simulink model "MPG_MG_PLL_orig"  (R2021b)
settings: Solver=VariableStepAuto  StartTime=0.0  StopTime=1  RelTol=1e-3
model workspace (MAT data in the model file):
  Ts : Simulink.Parameter (value not decoded)
  secondary_on : Simulink.Parameter (value not decoded)
values from neighbouring files (symbols this model uses):
  A = zeros(4,4)    [MPC_MG_script_raw_dmpc.m]    (also in MPG_MG_July.m = [0 1 1 1; 1 0 0 0; 1 0 0 0; 1 0 0 0]; MPG_MG_freq_script.m = ones(4) - eye(4); Script.m = [0 1 1 1 ; 1 0 1 1 ; 1 1 0 1 ; 1 1 1 0])
  C_f = 50e-6    (= 5e-05)    [Four_DG_MG_PrimaryOnlyScript.m]    (also in MPC_MG_script.m; MPC_MG_script_raw_dmpc.m; MPC_MG_secondary_script.m; MPG_MG_July.m)
  f_c = 5000    [Four_DG_MG_PrimaryOnlyScript.m]    (also in MPC_MG_script.m = 40000; MPC_MG_script_raw_dmpc.m = 40000; MPC_MG_secondary_script.m = 40000; MPG_MG_July.m = 50000)
  kL = 1e-5    (= 1e-05)    [Four_DG_MG_PrimaryOnlyScript.m]    (also in MPC_MG_script.m = 1e-08; MPC_MG_script_raw_dmpc.m = 1e-08; MPC_MG_secondary_script.m = 1e-07; MPG_MG_July.m = 1e-07)
  L_f = 1.35e-3    (= 0.00135)    [Four_DG_MG_PrimaryOnlyScript.m]    (also in MPC_MG_script.m; MPC_MG_script_raw_dmpc.m; MPC_MG_secondary_script.m; MPG_MG_July.m)
  L_in1 = 0.35e-3    (= 0.00035)    [Four_DG_MG_PrimaryOnlyScript.m]    (also in MPC_MG_script.m; MPC_MG_script_raw_dmpc.m; MPC_MG_secondary_script.m; MPG_MG_July.m)
  L_in2 = 0.35e-3    (= 0.00035)    [Four_DG_MG_PrimaryOnlyScript.m]    (also in MPC_MG_script.m; MPC_MG_script_raw_dmpc.m; MPC_MG_secondary_script.m; MPG_MG_July.m)
  L_in4 = 0.35e-3    (= 0.00035)    [Four_DG_MG_PrimaryOnlyScript.m]    (also in MPC_MG_script.m; MPC_MG_script_raw_dmpc.m; MPC_MG_secondary_script.m; MPG_MG_July.m)
  lambda1 = [30000 50000 90000 50000]'    [MPC_MG_script_raw_dmpc.m]    (also in MPG_MG_July.m = [4 4 4 4]'; MPG_MG_freq_script.m = [3 3 3 3]'; Script.m = [1 1 1 1]')
  lambda2 = [5 6 7 6]'    [MPC_MG_script_raw_dmpc.m]    (also in MPG_MG_July.m = [0.5e-2 0.5e-2 0.5e-2 0.5e-2]'; MPG_MG_freq_script.m = [1.1 1.9 1.5 1.2]'; Script.m = [0.8e-2 0.8e-2 0.8e-2 0.8e-2]')
  lambda3 = [80000 80000 900000 80000]'    [MPC_MG_script_raw_dmpc.m]    (also in MPG_MG_July.m = [1e-3 1e-3 1e-3 1e-3]'; MPG_MG_freq_script.m = [9e-4 1.2e-2 3e-3 3e-3]'; Script.m = [1.5e-3 1.5e-3 1.5e-3 1.5e-3]')
  LD_ref1 = 800e-6    (= 0.0008)    [Four_DG_MG_PrimaryOnlyScript.m]    (also in MPC_MG_script.m = 0.0003; MPC_MG_script_raw_dmpc.m = 0.0003; MPC_MG_secondary_script.m = 0.0001; MPG_MG_July.m = 0.0004)
  lo_co = 0.2    [Four_DG_MG_PrimaryOnlyScript.m]    (also in MPC_MG_script.m = 0.05; MPC_MG_script_raw_dmpc.m; MPC_MG_secondary_script.m = 0.08; MPG_MG_July.m = 0.15)
  m_p1 = 9.4e-5/droopDivide    (= 9.4e-05)    [Four_DG_MG_PrimaryOnlyScript.m]    (also in MPC_MG_script.m; MPC_MG_script_raw_dmpc.m; MPC_MG_secondary_script.m; MPG_MG_July.m)
  m_p2 = 9.4e-5/droopDivide    (= 9.4e-05)    [Four_DG_MG_PrimaryOnlyScript.m]    (also in MPC_MG_script.m; MPC_MG_script_raw_dmpc.m; MPC_MG_secondary_script.m; MPG_MG_July.m)
  m_p3 = 12.5e-5/droopDivide    (= 0.000125)    [Four_DG_MG_PrimaryOnlyScript.m]    (also in MPC_MG_script.m; MPC_MG_script_raw_dmpc.m; MPC_MG_secondary_script.m; MPG_MG_July.m)
  m_p4 = 12.5e-5/droopDivide    (= 0.000125)    [Four_DG_MG_PrimaryOnlyScript.m]    (also in MPC_MG_script.m; MPC_MG_script_raw_dmpc.m; MPC_MG_secondary_script.m; MPG_MG_July.m)
  N = 3    [MPG_MG_July.m]    (also in MPG_MG_freq_script.m = 2; Script.m = 5)
  n_q1 = 1.3e-3/droopDivide2    (= 0.00013)    [Four_DG_MG_PrimaryOnlyScript.m]    (also in MPC_MG_script.m; MPC_MG_script_raw_dmpc.m; MPC_MG_secondary_script.m; MPG_MG_July.m)
  n_q2 = 1.3e-3/droopDivide2    (= 0.00013)    [Four_DG_MG_PrimaryOnlyScript.m]    (also in MPC_MG_script.m; MPC_MG_script_raw_dmpc.m; MPC_MG_secondary_script.m; MPG_MG_July.m)
  n_q4 = 1.5e-3/droopDivide2    (= 0.00015)    [Four_DG_MG_PrimaryOnlyScript.m]    (also in MPC_MG_script.m; MPC_MG_script_raw_dmpc.m; MPC_MG_secondary_script.m; MPG_MG_July.m)
  Pmax = [45e3 45e3 37e3 37e3]'    [MPG_MG_July.m]    (also in MPG_MG_freq_script.m; Script.m)
  R_f = 0.1    [Four_DG_MG_PrimaryOnlyScript.m]    (also in MPC_MG_script.m; MPC_MG_script_raw_dmpc.m; MPC_MG_secondary_script.m; MPG_MG_July.m)
  R_in1 = 0.03    [Four_DG_MG_PrimaryOnlyScript.m]    (also in MPC_MG_script.m; MPC_MG_script_raw_dmpc.m; MPC_MG_secondary_script.m; MPG_MG_July.m)
  R_in2 = 0.03    [Four_DG_MG_PrimaryOnlyScript.m]    (also in MPC_MG_script.m; MPC_MG_script_raw_dmpc.m; MPC_MG_secondary_script.m; MPG_MG_July.m)
  R_in4 = 0.03    [Four_DG_MG_PrimaryOnlyScript.m]    (also in MPC_MG_script.m; MPC_MG_script_raw_dmpc.m; MPC_MG_secondary_script.m; MPG_MG_July.m)
  time_thresh = 0.6    [Four_DG_MG_PrimaryOnlyScript.m]    (also in MPC_MG_script_raw_dmpc.m = 1.5; MPC_MG_secondary_script.m = 2; MPG_MG_July.m = 0.5; MPG_MG_freq_script.m = 0.5)
  Ts = 10e-6    (= 1e-05)    [Four_DG_MG_PrimaryOnlyScript.m]    (also in MPC_MG_script.m; MPC_MG_script_raw_dmpc.m; MPC_MG_secondary_script.m; MPG_MG_July.m)
  Tsamp = 0.1    [MPG_MG_July.m]    (also in MPG_MG_freq_script.m; Script.m)
  V_nom = 220*sqrt(2)    [Four_DG_MG_PrimaryOnlyScript.m]    (also in MPC_MG_script.m; MPC_MG_script_raw_dmpc.m; MPC_MG_secondary_script.m; MPG_MG_July.m)
  Vdc = 600    [Four_DG_MG_PrimaryOnlyScript.m]    (also in MPC_MG_script.m; MPC_MG_script_raw_dmpc.m; MPC_MG_secondary_script.m; MPG_MG_July.m)
  w_c_high = 2*pi*50    (= 314.159265359)    [Four_DG_MG_PrimaryOnlyScript.m]    (also in MPC_MG_script.m; MPC_MG_script_raw_dmpc.m; MPC_MG_secondary_script.m; MPG_MG_July.m)
  w_nom = 2*pi*50    (= 314.159265359)    [Four_DG_MG_PrimaryOnlyScript.m]    (also in MPC_MG_script.m; MPC_MG_script_raw_dmpc.m; MPC_MG_secondary_script.m; MPG_MG_July.m)
undefined symbols (not defined in the file or in its folder): i
libraries: spsThreePhaseSeriesRLCBranchLib x18, spsabctodq0Lib x16, spsThreePhaseVIMeasurementLib x15, eeGeneralControl x15, dspswit3 x5, spsDCVoltageSourceLib x5, spsSeriesRLCBranchLib x5, spsTwoLevelConverterLib x5, slpidlib x5, spsAlphaBetaZerotodq0Lib x4, spsSecondOrderFilterLib x4, spsThreePhaseSeriesRLCLoadLib x2
(part 5 of 6)

== system MPG_MG_PLL_orig/Voltage Source Inverter 4/CDSC-PLL/DSC4/DSC_Beta ==
  Alpha : Inport
  Beta : Inport  Port=2
  Cos 2*pi/n : Subsystem
  Divide : Product  Inputs=*/
  Divide1 : Product  Inputs=*/
  Gain : Gain  Gain=1/2
  Product : Product
  Product1 : Product
  Sin 2*pi/n : Subsystem
  Sum1 : Sum  Inputs=+++
  T/n : Constant  Value=1/n
  T/n1 : Constant  Value=1/n
  Variable Transport Delay : VariableTransportDelay  VariableDelayType=Variable transport delay  MaximumDelay=10
  Variable Transport Delay1 : VariableTransportDelay  VariableDelayType=Variable transport delay  MaximumDelay=10
  Out : Outport  VectorParamsAs1DForOutWhenUnconnected=off
  wires:
  Gain/1 -> Out/1
  Sum1/1 -> Gain/1
  Beta/1 -> Variable Transport Delay/1, Sum1/1
  Alpha/1 -> Variable Transport Delay1/1
  Cos 2*pi/n/1(cos) -> Product/2
  Product/1 -> Sum1/2
  Variable Transport Delay/1 -> Product/1
  Variable Transport Delay1/1 -> Product1/1
  Product1/1 -> Sum1/3
  Sin 2*pi/n/1(sin) -> Product1/2
  T/n/1 -> Divide/1
  Divide/1 -> Variable Transport Delay/2
  [f_pll_c3] -> Divide/2
  T/n1/1 -> Divide1/1
  Divide1/1 -> Variable Transport Delay1/2
  [f_pll_c3] -> Divide1/2

== system MPG_MG_PLL_orig/Voltage Source Inverter 4/CDSC-PLL/DSC4/DSC_alpha ==
  Alpha : Inport
  Beta : Inport  Port=2
  Cos 2*pi/n : Subsystem
  Divide : Product  Inputs=*/
  Divide1 : Product  Inputs=*/
  Gain : Gain  Gain=1/2
  Product : Product
  Product1 : Product
  Sin 2*pi/n : Subsystem
  Sum1 : Sum  Inputs=++-
  T/n : Constant  Value=1/n
  T/n1 : Constant  Value=1/n
  Variable Transport Delay : VariableTransportDelay  VariableDelayType=Variable transport delay  MaximumDelay=10
  Variable Transport Delay1 : VariableTransportDelay  VariableDelayType=Variable transport delay  MaximumDelay=10
  Out : Outport  VectorParamsAs1DForOutWhenUnconnected=off
  wires:
  Sum1/1 -> Gain/1
  Gain/1 -> Out/1
  Sin 2*pi/n/1(sin) -> Product1/2
  Beta/1 -> Variable Transport Delay1/1
  Product1/1 -> Sum1/3
  Variable Transport Delay1/1 -> Product1/1
  Alpha/1 -> Variable Transport Delay/1, Sum1/1
  Variable Transport Delay/1 -> Product/1
  Product/1 -> Sum1/2
  Cos 2*pi/n/1(cos) -> Product/2
  T/n1/1 -> Divide/1
  Divide/1 -> Variable Transport Delay1/2
  [f_pll_c3] -> Divide/2
  T/n/1 -> Divide1/1
  Divide1/1 -> Variable Transport Delay/2
  [f_pll_c3] -> Divide1/2

== system MPG_MG_PLL_orig/Voltage Source Inverter 4/CDSC-PLL/DSC8/DSC_Beta ==
  Alpha : Inport
  Beta : Inport  Port=2
  Cos 2*pi/n : Subsystem
  Divide : Product  Inputs=*/
  Divide1 : Product  Inputs=*/
  Gain : Gain  Gain=1/2
  Product : Product
  Product1 : Product
  Sin 2*pi/n : Subsystem
  Sum1 : Sum  Inputs=+++
  T/n : Constant  Value=1/n
  T/n1 : Constant  Value=1/n
  Variable Transport Delay : VariableTransportDelay  VariableDelayType=Variable transport delay  MaximumDelay=10
  Variable Transport Delay1 : VariableTransportDelay  VariableDelayType=Variable transport delay  MaximumDelay=10
  Out : Outport  VectorParamsAs1DForOutWhenUnconnected=off
  wires:
  Sin 2*pi/n/1(sin) -> Product1/2
  Product1/1 -> Sum1/3
  Variable Transport Delay1/1 -> Product1/1
  Variable Transport Delay/1 -> Product/1
  Product/1 -> Sum1/2
  Cos 2*pi/n/1(cos) -> Product/2
  Alpha/1 -> Variable Transport Delay1/1
  Beta/1 -> Sum1/1, Variable Transport Delay/1
  Sum1/1 -> Gain/1
  Gain/1 -> Out/1
  T/n/1 -> Divide/1
  Divide/1 -> Variable Transport Delay/2
  [f_pll_c3] -> Divide/2
  T/n1/1 -> Divide1/1
  Divide1/1 -> Variable Transport Delay1/2
  [f_pll_c3] -> Divide1/2

== system MPG_MG_PLL_orig/Voltage Source Inverter 4/CDSC-PLL/DSC8/DSC_alpha ==
  Alpha : Inport
  Beta : Inport  Port=2
  Cos 2*pi/n : Subsystem
  Divide : Product  Inputs=*/
  Divide1 : Product  Inputs=*/
  Gain : Gain  Gain=1/2
  Product : Product
  Product1 : Product
  Sin 2*pi/n : Subsystem
  Sum1 : Sum  Inputs=++-
  T/n : Constant  Value=1/n
  T/n1 : Constant  Value=1/n
  Variable Transport Delay : VariableTransportDelay  VariableDelayType=Variable transport delay  MaximumDelay=10
  Variable Transport Delay1 : VariableTransportDelay  VariableDelayType=Variable transport delay  MaximumDelay=10
  Out : Outport  VectorParamsAs1DForOutWhenUnconnected=off
  wires:
  Cos 2*pi/n/1(cos) -> Product/2
  Product/1 -> Sum1/2
  Variable Transport Delay/1 -> Product/1
  Alpha/1 -> Variable Transport Delay/1, Sum1/1
  Variable Transport Delay1/1 -> Product1/1
  Product1/1 -> Sum1/3
  Beta/1 -> Variable Transport Delay1/1
  Sin 2*pi/n/1(sin) -> Product1/2
  Gain/1 -> Out/1
  Sum1/1 -> Gain/1
  T/n/1 -> Divide/1
  Divide/1 -> Variable Transport Delay/2
  [f_pll_c3] -> Divide/2
  T/n1/1 -> Divide1/1
  Divide1/1 -> Variable Transport Delay1/2
  [f_pll_c3] -> Divide1/2

== system MPG_MG_PLL_orig/Voltage Source Inverter 4/CDSC-PLL/SRF-PLL1/Al_Be_0 to dq0 ==
  Al_Be_0 : Inport
  wt : Inport  Port=2
  Fcn : Fcn  Expr=u[1]*cos(u[4]) + u[2]*sin(u[4])
  Fcn1 : Fcn  Expr=-u[1]*sin(u[4]) + u[2]*cos(u[4])
  Fcn2 : Fcn  Expr=u[3]
  Mux1 : Mux  Inputs=[3 1]
  Mux2 : Mux  Inputs=3
  dq0 : Outport  VectorParamsAs1DForOutWhenUnconnected=off
  wires:
  Mux1/1 -> Fcn/1, Fcn2/1, Fcn1/1
  Fcn1/1 -> Mux2/2
  wt/1 -> Mux1/2
  Mux2/1 -> dq0/1
  Al_Be_0/1 -> Mux1/1
  Fcn2/1 -> Mux2/3
  Fcn/1 -> Mux2/1

== system MPG_MG_PLL_orig/Voltage Source Inverter 5/CDSC-PLL/DSC16/DSC_Beta ==
  Alpha : Inport
  Beta : Inport  Port=2
  Cos 2*pi/n : Subsystem
  Divide : Product  Inputs=*/
  Divide1 : Product  Inputs=*/
  Gain : Gain  Gain=1/2
  Product : Product
  Product1 : Product
  Sin 2*pi/n : Subsystem
  Sum1 : Sum  Inputs=+++
  T/n : Constant  Value=1/n
  T/n1 : Constant  Value=1/n
  Variable Transport Delay : VariableTransportDelay  VariableDelayType=Variable transport delay  MaximumDelay=10
  Variable Transport Delay1 : VariableTransportDelay  VariableDelayType=Variable transport delay  MaximumDelay=10
  Out : Outport  VectorParamsAs1DForOutWhenUnconnected=off
  wires:
  Gain/1 -> Out/1
  Sum1/1 -> Gain/1
  Beta/1 -> Variable Transport Delay/1, Sum1/1
  Alpha/1 -> Variable Transport Delay1/1
  Cos 2*pi/n/1(cos) -> Product/2
  Product/1 -> Sum1/2
  Variable Transport Delay/1 -> Product/1
  Variable Transport Delay1/1 -> Product1/1
  Product1/1 -> Sum1/3
  Sin 2*pi/n/1(sin) -> Product1/2
  T/n/1 -> Divide/1
  Divide/1 -> Variable Transport Delay/2
  [f_pll_c3] -> Divide/2
  T/n1/1 -> Divide1/1
  Divide1/1 -> Variable Transport Delay1/2
  [f_pll_c3] -> Divide1/2

== system MPG_MG_PLL_orig/Voltage Source Inverter 5/CDSC-PLL/DSC16/DSC_alpha ==
  Alpha : Inport
  Beta : Inport  Port=2
  Cos 2*pi/n : Subsystem
  Divide : Product  Inputs=*/
  Divide1 : Product  Inputs=*/
  Gain : Gain  Gain=1/2
  Product : Product
  Product1 : Product
  Sin 2*pi/n : Subsystem
  Sum1 : Sum  Inputs=++-
  T/n : Constant  Value=1/n
  T/n1 : Constant  Value=1/n
  Variable Transport Delay : VariableTransportDelay  VariableDelayType=Variable transport delay  MaximumDelay=10
  Variable Transport Delay1 : VariableTransportDelay  VariableDelayType=Variable transport delay  MaximumDelay=10
  Out : Outport  VectorParamsAs1DForOutWhenUnconnected=off
  wires:
  Sum1/1 -> Gain/1
  Gain/1 -> Out/1
  Sin 2*pi/n/1(sin) -> Product1/2
  Beta/1 -> Variable Transport Delay1/1
  Product1/1 -> Sum1/3
  Variable Transport Delay1/1 -> Product1/1
  Alpha/1 -> Variable Transport Delay/1, Sum1/1
  Variable Transport Delay/1 -> Product/1
  Product/1 -> Sum1/2
  Cos 2*pi/n/1(cos) -> Product/2
  T/n/1 -> Divide/1
  Divide/1 -> Variable Transport Delay/2
  [f_pll_c3] -> Divide/2
  T/n1/1 -> Divide1/1
  Divide1/1 -> Variable Transport Delay1/2
  [f_pll_c3] -> Divide1/2

== system MPG_MG_PLL_orig/Voltage Source Inverter 5/CDSC-PLL/DSC2/DSC_Beta ==
  Alpha : Inport
  Beta : Inport  Port=2
  Cos 2*pi/n : Subsystem
  Divide : Product  Inputs=*/
  Divide1 : Product  Inputs=*/
  Gain : Gain  Gain=1/2
  Product : Product
  Product1 : Product
  Sin 2*pi/n : Subsystem
  Sum1 : Sum  Inputs=+++
  T/n : Constant  Value=1/n
  T/n1 : Constant  Value=1/n
  Variable Transport Delay : VariableTransportDelay  VariableDelayType=Variable transport delay  MaximumDelay=10
  Variable Transport Delay1 : VariableTransportDelay  VariableDelayType=Variable transport delay  MaximumDelay=10
  Out : Outport  VectorParamsAs1DForOutWhenUnconnected=off
  wires:
  Sin 2*pi/n/1(sin) -> Product1/2
  Product1/1 -> Sum1/3
  Variable Transport Delay1/1 -> Product1/1
  Variable Transport Delay/1 -> Product/1
  Product/1 -> Sum1/2
  Cos 2*pi/n/1(cos) -> Product/2
  Alpha/1 -> Variable Transport Delay1/1
  Beta/1 -> Sum1/1, Variable Transport Delay/1
  Sum1/1 -> Gain/1
  Gain/1 -> Out/1
  T/n1/1 -> Divide/1
  Divide/1 -> Variable Transport Delay1/2
  [f_pll_c3] -> Divide/2
  T/n/1 -> Divide1/1
  Divide1/1 -> Variable Transport Delay/2
  [f_pll_c3] -> Divide1/2

== system MPG_MG_PLL_orig/Voltage Source Inverter 5/CDSC-PLL/DSC2/DSC_alpha ==
  Alpha : Inport
  Beta : Inport  Port=2
  Cos 2*pi/n : Subsystem
  Divide : Product  Inputs=*/
  Divide1 : Product  Inputs=*/
  Gain : Gain  Gain=1/2
  Product : Product
  Product1 : Product
  Sin 2*pi/n : Subsystem
  Sum1 : Sum  Inputs=++-
  T/n : Constant  Value=1/n
  T/n. : Constant  Value=1/n
  Variable Transport Delay : VariableTransportDelay  VariableDelayType=Variable transport delay  MaximumDelay=10
  Variable Transport Delay1 : VariableTransportDelay  VariableDelayType=Variable transport delay  MaximumDelay=10
  Out : Outport  VectorParamsAs1DForOutWhenUnconnected=off
  wires:
  Cos 2*pi/n/1(cos) -> Product/2
  Product/1 -> Sum1/2
  Variable Transport Delay/1 -> Product/1
  Alpha/1 -> Variable Transport Delay/1, Sum1/1
  Variable Transport Delay1/1 -> Product1/1
  Product1/1 -> Sum1/3
  Beta/1 -> Variable Transport Delay1/1
  Sin 2*pi/n/1(sin) -> Product1/2
  Gain/1 -> Out/1
  Sum1/1 -> Gain/1
  T/n/1 -> Divide/1
  Divide/1 -> Variable Transport Delay/2
  [f_pll_c3] -> Divide/2
  Divide1/1 -> Variable Transport Delay1/2
  T/n./1 -> Divide1/1
  [f_pll_c3] -> Divide1/2

== system MPG_MG_PLL_orig/Voltage Source Inverter 5/CDSC-PLL/DSC4/DSC_Beta ==
  Alpha : Inport
  Beta : Inport  Port=2
  Cos 2*pi/n : Subsystem
  Divide : Product  Inputs=*/
  Divide1 : Product  Inputs=*/
  Gain : Gain  Gain=1/2
  Product : Product
  Product1 : Product
  Sin 2*pi/n : Subsystem
  Sum1 : Sum  Inputs=+++
  T/n : Constant  Value=1/n
  T/n1 : Constant  Value=1/n
  Variable Transport Delay : VariableTransportDelay  VariableDelayType=Variable transport delay  MaximumDelay=10
  Variable Transport Delay1 : VariableTransportDelay  VariableDelayType=Variable transport delay  MaximumDelay=10
  Out : Outport  VectorParamsAs1DForOutWhenUnconnected=off
  wires:
  Gain/1 -> Out/1
  Sum1/1 -> Gain/1
  Beta/1 -> Variable Transport Delay/1, Sum1/1
  Alpha/1 -> Variable Transport Delay1/1
  Cos 2*pi/n/1(cos) -> Product/2
  Product/1 -> Sum1/2
  Variable Transport Delay/1 -> Product/1
  Variable Transport Delay1/1 -> Product1/1
  Product1/1 -> Sum1/3
  Sin 2*pi/n/1(sin) -> Product1/2
  T/n/1 -> Divide/1
  Divide/1 -> Variable Transport Delay/2
  [f_pll_c3] -> Divide/2
  T/n1/1 -> Divide1/1
  Divide1/1 -> Variable Transport Delay1/2
  [f_pll_c3] -> Divide1/2

== system MPG_MG_PLL_orig/Voltage Source Inverter 5/CDSC-PLL/DSC4/DSC_alpha ==
  Alpha : Inport
  Beta : Inport  Port=2
  Cos 2*pi/n : Subsystem
  Divide : Product  Inputs=*/
  Divide1 : Product  Inputs=*/
  Gain : Gain  Gain=1/2
  Product : Product
  Product1 : Product
  Sin 2*pi/n : Subsystem
  Sum1 : Sum  Inputs=++-
  T/n : Constant  Value=1/n
  T/n1 : Constant  Value=1/n
  Variable Transport Delay : VariableTransportDelay  VariableDelayType=Variable transport delay  MaximumDelay=10
  Variable Transport Delay1 : VariableTransportDelay  VariableDelayType=Variable transport delay  MaximumDelay=10
  Out : Outport  VectorParamsAs1DForOutWhenUnconnected=off
  wires:
  Sum1/1 -> Gain/1
  Gain/1 -> Out/1
  Sin 2*pi/n/1(sin) -> Product1/2
  Beta/1 -> Variable Transport Delay1/1
  Product1/1 -> Sum1/3
  Variable Transport Delay1/1 -> Product1/1
  Alpha/1 -> Variable Transport Delay/1, Sum1/1
  Variable Transport Delay/1 -> Product/1
  Product/1 -> Sum1/2
  Cos 2*pi/n/1(cos) -> Product/2
  T/n1/1 -> Divide/1
  Divide/1 -> Variable Transport Delay1/2
  [f_pll_c3] -> Divide/2
  T/n/1 -> Divide1/1
  Divide1/1 -> Variable Transport Delay/2
  [f_pll_c3] -> Divide1/2

== system MPG_MG_PLL_orig/Voltage Source Inverter 5/CDSC-PLL/DSC8/DSC_Beta ==
  Alpha : Inport
  Beta : Inport  Port=2
  Cos 2*pi/n : Subsystem
  Divide : Product  Inputs=*/
  Divide1 : Product  Inputs=*/
  Gain : Gain  Gain=1/2
  Product : Product
  Product1 : Product
  Sin 2*pi/n : Subsystem
  Sum1 : Sum  Inputs=+++
  T/n : Constant  Value=1/n
  T/n1 : Constant  Value=1/n
  Variable Transport Delay : VariableTransportDelay  VariableDelayType=Variable transport delay  MaximumDelay=10
  Variable Transport Delay1 : VariableTransportDelay  VariableDelayType=Variable transport delay  MaximumDelay=10
  Out : Outport  VectorParamsAs1DForOutWhenUnconnected=off
  wires:
  Sin 2*pi/n/1(sin) -> Product1/2
  Product1/1 -> Sum1/3
  Variable Transport Delay1/1 -> Product1/1
  Variable Transport Delay/1 -> Product/1
  Product/1 -> Sum1/2
  Cos 2*pi/n/1(cos) -> Product/2
  Alpha/1 -> Variable Transport Delay1/1
  Beta/1 -> Sum1/1, Variable Transport Delay/1
  Sum1/1 -> Gain/1
  Gain/1 -> Out/1
  T/n/1 -> Divide/1
  Divide/1 -> Variable Transport Delay/2
  [f_pll_c3] -> Divide/2
  T/n1/1 -> Divide1/1
  Divide1/1 -> Variable Transport Delay1/2
  [f_pll_c3] -> Divide1/2

== system MPG_MG_PLL_orig/Voltage Source Inverter 5/CDSC-PLL/DSC8/DSC_alpha ==
  Alpha : Inport
  Beta : Inport  Port=2
  Cos 2*pi/n : Subsystem
  Divide : Product  Inputs=*/
  Divide1 : Product  Inputs=*/
  Gain : Gain  Gain=1/2
  Product : Product
  Product1 : Product
  Sin 2*pi/n : Subsystem
  Sum1 : Sum  Inputs=++-
  T/n : Constant  Value=1/n
  T/n1 : Constant  Value=1/n
  Variable Transport Delay : VariableTransportDelay  VariableDelayType=Variable transport delay  MaximumDelay=10
  Variable Transport Delay1 : VariableTransportDelay  VariableDelayType=Variable transport delay  MaximumDelay=10
  Out : Outport  VectorParamsAs1DForOutWhenUnconnected=off
  wires:
  Cos 2*pi/n/1(cos) -> Product/2
  Product/1 -> Sum1/2
  Variable Transport Delay/1 -> Product/1
  Alpha/1 -> Variable Transport Delay/1, Sum1/1
  Variable Transport Delay1/1 -> Product1/1
  Product1/1 -> Sum1/3
  Beta/1 -> Variable Transport Delay1/1
  Sin 2*pi/n/1(sin) -> Product1/2
  Gain/1 -> Out/1
  Sum1/1 -> Gain/1
  T/n/1 -> Divide/1
  Divide/1 -> Variable Transport Delay/2
  [f_pll_c3] -> Divide/2
  T/n1/1 -> Divide1/1
  Divide1/1 -> Variable Transport Delay1/2
  [f_pll_c3] -> Divide1/2

== system MPG_MG_PLL_orig/Voltage Source Inverter 5/CDSC-PLL/SRF-PLL1/Al_Be_0 to dq0 ==
  Al_Be_0 : Inport
  wt : Inport  Port=2
  Fcn : Fcn  Expr=u[1]*cos(u[4]) + u[2]*sin(u[4])
  Fcn1 : Fcn  Expr=-u[1]*sin(u[4]) + u[2]*cos(u[4])
  Fcn2 : Fcn  Expr=u[3]
  Mux1 : Mux  Inputs=[3 1]
  Mux2 : Mux  Inputs=3
  dq0 : Outport  VectorParamsAs1DForOutWhenUnconnected=off
  wires:
  Mux1/1 -> Fcn/1, Fcn2/1, Fcn1/1
  Fcn1/1 -> Mux2/2
  wt/1 -> Mux1/2
  Mux2/1 -> dq0/1
  Al_Be_0/1 -> Mux1/1
  Fcn2/1 -> Mux2/3
  Fcn/1 -> Mux2/1

== system MPG_MG_PLL_orig/Voltage Source Inverter 2/CDSC-PLL/DSC16/DSC_Beta/Cos 2*pi//n ==
  note: 2*pi*hr/n
  Constant : Constant  Value=2*pi/n
  Trigonometric Function : Trigonometry  Operator=cos
  cos : Outport  VectorParamsAs1DForOutWhenUnconnected=off
  wires:
  Trigonometric Function/1 -> cos/1
  Constant/1 -> Trigonometric Function/1

== system MPG_MG_PLL_orig/Voltage Source Inverter 2/CDSC-PLL/DSC16/DSC_Beta/Sin 2*pi//n ==
  note: 2*pi/n
  Constant : Constant  Value=2*pi/n
  Trigonometric Function : Trigonometry
  sin : Outport  VectorParamsAs1DForOutWhenUnconnected=off
  wires:
  Trigonometric Function/1 -> sin/1
  Constant/1 -> Trigonometric Function/1

== system MPG_MG_PLL_orig/Voltage Source Inverter 2/CDSC-PLL/DSC16/DSC_alpha/Cos 2*pi//n ==
  note: 2*pi*hr/n
  Constant : Constant  Value=2*pi/n
  Trigonometric Function : Trigonometry  Operator=cos
  cos : Outport  VectorParamsAs1DForOutWhenUnconnected=off
  wires:
  Trigonometric Function/1 -> cos/1
  Constant/1 -> Trigonometric Function/1

== system MPG_MG_PLL_orig/Voltage Source Inverter 2/CDSC-PLL/DSC16/DSC_alpha/Sin 2*pi//n ==
  note: 2*pi/n
  Constant : Constant  Value=2*pi/n
  Trigonometric Function : Trigonometry
  sin : Outport  VectorParamsAs1DForOutWhenUnconnected=off
  wires:
  Trigonometric Function/1 -> sin/1
  Constant/1 -> Trigonometric Function/1

== system MPG_MG_PLL_orig/Voltage Source Inverter 2/CDSC-PLL/DSC2/DSC_Beta/Cos 2*pi//n ==
  note: 2*pi*hr/n
  Constant : Constant  Value=2*pi/n
  Trigonometric Function : Trigonometry  Operator=cos
  cos : Outport  VectorParamsAs1DForOutWhenUnconnected=off
  wires:
  Trigonometric Function/1 -> cos/1
  Constant/1 -> Trigonometric Function/1

== system MPG_MG_PLL_orig/Voltage Source Inverter 2/CDSC-PLL/DSC2/DSC_Beta/Sin 2*pi//n ==
  note: 2*pi/n
  Constant : Constant  Value=2*pi/n
  Trigonometric Function : Trigonometry
  sin : Outport  VectorParamsAs1DForOutWhenUnconnected=off
  wires:
  Trigonometric Function/1 -> sin/1
  Constant/1 -> Trigonometric Function/1

== system MPG_MG_PLL_orig/Voltage Source Inverter 2/CDSC-PLL/DSC2/DSC_alpha/Cos 2*pi//n ==
  note: 2*pi*hr/n
  Constant : Constant  Value=2*pi/n
  Trigonometric Function : Trigonometry  Operator=cos
  cos : Outport  VectorParamsAs1DForOutWhenUnconnected=off
  wires:
  Trigonometric Function/1 -> cos/1
  Constant/1 -> Trigonometric Function/1

== system MPG_MG_PLL_orig/Voltage Source Inverter 2/CDSC-PLL/DSC2/DSC_alpha/Sin 2*pi//n ==
  note: 2*pi/n
  Constant : Constant  Value=2*pi/n
  Trigonometric Function : Trigonometry
  sin : Outport  VectorParamsAs1DForOutWhenUnconnected=off
  wires:
  Trigonometric Function/1 -> sin/1
  Constant/1 -> Trigonometric Function/1

== system MPG_MG_PLL_orig/Voltage Source Inverter 2/CDSC-PLL/DSC4/DSC_Beta/Cos 2*pi//n ==
  note: 2*pi*hr/n
  Constant : Constant  Value=2*pi/n
  Trigonometric Function : Trigonometry  Operator=cos
  cos : Outport  VectorParamsAs1DForOutWhenUnconnected=off
  wires:
  Trigonometric Function/1 -> cos/1
  Constant/1 -> Trigonometric Function/1

== system MPG_MG_PLL_orig/Voltage Source Inverter 2/CDSC-PLL/DSC4/DSC_Beta/Sin 2*pi//n ==
  note: 2*pi/n
  Constant : Constant  Value=2*pi/n
  Trigonometric Function : Trigonometry
  sin : Outport  VectorParamsAs1DForOutWhenUnconnected=off
  wires:
  Trigonometric Function/1 -> sin/1
  Constant/1 -> Trigonometric Function/1

== system MPG_MG_PLL_orig/Voltage Source Inverter 2/CDSC-PLL/DSC4/DSC_alpha/Cos 2*pi//n ==
  note: 2*pi*hr/n
  Constant : Constant  Value=2*pi/n
  Trigonometric Function : Trigonometry  Operator=cos
  cos : Outport  VectorParamsAs1DForOutWhenUnconnected=off
  wires:
  Trigonometric Function/1 -> cos/1
  Constant/1 -> Trigonometric Function/1

== system MPG_MG_PLL_orig/Voltage Source Inverter 2/CDSC-PLL/DSC4/DSC_alpha/Sin 2*pi//n ==
  note: 2*pi/n
  Constant : Constant  Value=2*pi/n
  Trigonometric Function : Trigonometry
  sin : Outport  VectorParamsAs1DForOutWhenUnconnected=off
  wires:
  Trigonometric Function/1 -> sin/1
  Constant/1 -> Trigonometric Function/1

== system MPG_MG_PLL_orig/Voltage Source Inverter 2/CDSC-PLL/DSC8/DSC_Beta/Cos 2*pi//n ==
  note: 2*pi*hr/n
  Constant : Constant  Value=2*pi/n
  Trigonometric Function : Trigonometry  Operator=cos
  cos : Outport  VectorParamsAs1DForOutWhenUnconnected=off
  wires:
  Trigonometric Function/1 -> cos/1
  Constant/1 -> Trigonometric Function/1

== system MPG_MG_PLL_orig/Voltage Source Inverter 2/CDSC-PLL/DSC8/DSC_Beta/Sin 2*pi//n ==
  note: 2*pi/n
  Constant : Constant  Value=2*pi/n
  Trigonometric Function : Trigonometry
  sin : Outport  VectorParamsAs1DForOutWhenUnconnected=off
  wires:
  Trigonometric Function/1 -> sin/1
  Constant/1 -> Trigonometric Function/1

== system MPG_MG_PLL_orig/Voltage Source Inverter 2/CDSC-PLL/DSC8/DSC_alpha/Cos 2*pi//n ==
  note: 2*pi*hr/n
  Constant : Constant  Value=2*pi/n
  Trigonometric Function : Trigonometry  Operator=cos
  cos : Outport  VectorParamsAs1DForOutWhenUnconnected=off
  wires:
  Trigonometric Function/1 -> cos/1
  Constant/1 -> Trigonometric Function/1

== system MPG_MG_PLL_orig/Voltage Source Inverter 2/CDSC-PLL/DSC8/DSC_alpha/Sin 2*pi//n ==
  note: 2*pi/n
  Constant : Constant  Value=2*pi/n
  Trigonometric Function : Trigonometry
  sin : Outport  VectorParamsAs1DForOutWhenUnconnected=off
  wires:
  Trigonometric Function/1 -> sin/1
  Constant/1 -> Trigonometric Function/1

== system MPG_MG_PLL_orig/Voltage Source Inverter 3/CDSC-PLL/DSC16/DSC_Beta/Cos 2*pi//n ==
  note: 2*pi*hr/n
  Constant : Constant  Value=2*pi/n
  Trigonometric Function : Trigonometry  Operator=cos
  cos : Outport  VectorParamsAs1DForOutWhenUnconnected=off
  wires:
  Trigonometric Function/1 -> cos/1
  Constant/1 -> Trigonometric Function/1

== system MPG_MG_PLL_orig/Voltage Source Inverter 3/CDSC-PLL/DSC16/DSC_Beta/Sin 2*pi//n ==
  note: 2*pi/n
  Constant : Constant  Value=2*pi/n
  Trigonometric Function : Trigonometry
  sin : Outport  VectorParamsAs1DForOutWhenUnconnected=off
  wires:
  Trigonometric Function/1 -> sin/1
  Constant/1 -> Trigonometric Function/1

== system MPG_MG_PLL_orig/Voltage Source Inverter 3/CDSC-PLL/DSC16/DSC_alpha/Cos 2*pi//n ==
  note: 2*pi*hr/n
  Constant : Constant  Value=2*pi/n
  Trigonometric Function : Trigonometry  Operator=cos
  cos : Outport  VectorParamsAs1DForOutWhenUnconnected=off
  wires:
  Trigonometric Function/1 -> cos/1
  Constant/1 -> Trigonometric Function/1

== system MPG_MG_PLL_orig/Voltage Source Inverter 3/CDSC-PLL/DSC16/DSC_alpha/Sin 2*pi//n ==
  note: 2*pi/n
  Constant : Constant  Value=2*pi/n
  Trigonometric Function : Trigonometry
  sin : Outport  VectorParamsAs1DForOutWhenUnconnected=off
  wires:
  Trigonometric Function/1 -> sin/1
  Constant/1 -> Trigonometric Function/1

== system MPG_MG_PLL_orig/Voltage Source Inverter 3/CDSC-PLL/DSC2/DSC_Beta/Cos 2*pi//n ==
  note: 2*pi*hr/n
  Constant : Constant  Value=2*pi/n
  Trigonometric Function : Trigonometry  Operator=cos
  cos : Outport  VectorParamsAs1DForOutWhenUnconnected=off
  wires:
  Trigonometric Function/1 -> cos/1
  Constant/1 -> Trigonometric Function/1

== system MPG_MG_PLL_orig/Voltage Source Inverter 3/CDSC-PLL/DSC2/DSC_Beta/Sin 2*pi//n ==
  note: 2*pi/n
  Constant : Constant  Value=2*pi/n
  Trigonometric Function : Trigonometry
  sin : Outport  VectorParamsAs1DForOutWhenUnconnected=off
  wires:
  Trigonometric Function/1 -> sin/1
  Constant/1 -> Trigonometric Function/1

== system MPG_MG_PLL_orig/Voltage Source Inverter 3/CDSC-PLL/DSC2/DSC_alpha/Cos 2*pi//n ==
  note: 2*pi*hr/n
  Constant : Constant  Value=2*pi/n
  Trigonometric Function : Trigonometry  Operator=cos
  cos : Outport  VectorParamsAs1DForOutWhenUnconnected=off
  wires:
  Trigonometric Function/1 -> cos/1
  Constant/1 -> Trigonometric Function/1

== system MPG_MG_PLL_orig/Voltage Source Inverter 3/CDSC-PLL/DSC2/DSC_alpha/Sin 2*pi//n ==
  note: 2*pi/n
  Constant : Constant  Value=2*pi/n
  Trigonometric Function : Trigonometry
  sin : Outport  VectorParamsAs1DForOutWhenUnconnected=off
  wires:
  Trigonometric Function/1 -> sin/1
  Constant/1 -> Trigonometric Function/1

== system MPG_MG_PLL_orig/Voltage Source Inverter 3/CDSC-PLL/DSC4/DSC_Beta/Cos 2*pi//n ==
  note: 2*pi*hr/n
  Constant : Constant  Value=2*pi/n
  Trigonometric Function : Trigonometry  Operator=cos
  cos : Outport  VectorParamsAs1DForOutWhenUnconnected=off
  wires:
  Trigonometric Function/1 -> cos/1
  Constant/1 -> Trigonometric Function/1

== system MPG_MG_PLL_orig/Voltage Source Inverter 3/CDSC-PLL/DSC4/DSC_Beta/Sin 2*pi//n ==
  note: 2*pi/n
  Constant : Constant  Value=2*pi/n
  Trigonometric Function : Trigonometry
  sin : Outport  VectorParamsAs1DForOutWhenUnconnected=off
  wires:
  Trigonometric Function/1 -> sin/1
  Constant/1 -> Trigonometric Function/1

== system MPG_MG_PLL_orig/Voltage Source Inverter 3/CDSC-PLL/DSC4/DSC_alpha/Cos 2*pi//n ==
  note: 2*pi*hr/n
  Constant : Constant  Value=2*pi/n
  Trigonometric Function : Trigonometry  Operator=cos
  cos : Outport  VectorParamsAs1DForOutWhenUnconnected=off
  wires:
  Trigonometric Function/1 -> cos/1
  Constant/1 -> Trigonometric Function/1

== system MPG_MG_PLL_orig/Voltage Source Inverter 3/CDSC-PLL/DSC4/DSC_alpha/Sin 2*pi//n ==
  note: 2*pi/n
  Constant : Constant  Value=2*pi/n
  Trigonometric Function : Trigonometry
  sin : Outport  VectorParamsAs1DForOutWhenUnconnected=off
  wires:
  Trigonometric Function/1 -> sin/1
  Constant/1 -> Trigonometric Function/1

== system MPG_MG_PLL_orig/Voltage Source Inverter 3/CDSC-PLL/DSC8/DSC_Beta/Cos 2*pi//n ==
  note: 2*pi*hr/n
  Constant : Constant  Value=2*pi/n
  Trigonometric Function : Trigonometry  Operator=cos
  cos : Outport  VectorParamsAs1DForOutWhenUnconnected=off
  wires:
  Trigonometric Function/1 -> cos/1
  Constant/1 -> Trigonometric Function/1

== system MPG_MG_PLL_orig/Voltage Source Inverter 3/CDSC-PLL/DSC8/DSC_Beta/Sin 2*pi//n ==
  note: 2*pi/n
  Constant : Constant  Value=2*pi/n
  Trigonometric Function : Trigonometry
  sin : Outport  VectorParamsAs1DForOutWhenUnconnected=off
  wires:
  Trigonometric Function/1 -> sin/1
  Constant/1 -> Trigonometric Function/1

== system MPG_MG_PLL_orig/Voltage Source Inverter 3/CDSC-PLL/DSC8/DSC_alpha/Cos 2*pi//n ==
  note: 2*pi*hr/n
  Constant : Constant  Value=2*pi/n
  Trigonometric Function : Trigonometry  Operator=cos
  cos : Outport  VectorParamsAs1DForOutWhenUnconnected=off
  wires:
  Trigonometric Function/1 -> cos/1
  Constant/1 -> Trigonometric Function/1

== system MPG_MG_PLL_orig/Voltage Source Inverter 3/CDSC-PLL/DSC8/DSC_alpha/Sin 2*pi//n ==
  note: 2*pi/n
  Constant : Constant  Value=2*pi/n
  Trigonometric Function : Trigonometry
  sin : Outport  VectorParamsAs1DForOutWhenUnconnected=off
  wires:
  Trigonometric Function/1 -> sin/1
  Constant/1 -> Trigonometric Function/1

== system MPG_MG_PLL_orig/Voltage Source Inverter 4/CDSC-PLL/DSC16/DSC_Beta/Cos 2*pi//n ==
  note: 2*pi*hr/n
  Constant : Constant  Value=2*pi/n
  Trigonometric Function : Trigonometry  Operator=cos
  cos : Outport  VectorParamsAs1DForOutWhenUnconnected=off
  wires:
  Trigonometric Function/1 -> cos/1
  Constant/1 -> Trigonometric Function/1

== system MPG_MG_PLL_orig/Voltage Source Inverter 4/CDSC-PLL/DSC16/DSC_Beta/Sin 2*pi//n ==
  note: 2*pi/n
  Constant : Constant  Value=2*pi/n
  Trigonometric Function : Trigonometry
  sin : Outport  VectorParamsAs1DForOutWhenUnconnected=off
  wires:
  Trigonometric Function/1 -> sin/1
  Constant/1 -> Trigonometric Function/1

== system MPG_MG_PLL_orig/Voltage Source Inverter 4/CDSC-PLL/DSC16/DSC_alpha/Cos 2*pi//n ==
  note: 2*pi*hr/n
  Constant : Constant  Value=2*pi/n
  Trigonometric Function : Trigonometry  Operator=cos
  cos : Outport  VectorParamsAs1DForOutWhenUnconnected=off
  wires:
  Trigonometric Function/1 -> cos/1
  Constant/1 -> Trigonometric Function/1

== system MPG_MG_PLL_orig/Voltage Source Inverter 4/CDSC-PLL/DSC16/DSC_alpha/Sin 2*pi//n ==
  note: 2*pi/n
  Constant : Constant  Value=2*pi/n
  Trigonometric Function : Trigonometry
  sin : Outport  VectorParamsAs1DForOutWhenUnconnected=off
  wires:
  Trigonometric Function/1 -> sin/1
  Constant/1 -> Trigonometric Function/1

== system MPG_MG_PLL_orig/Voltage Source Inverter 4/CDSC-PLL/DSC2/DSC_Beta/Cos 2*pi//n ==
  note: 2*pi*hr/n
  Constant : Constant  Value=2*pi/n
  Trigonometric Function : Trigonometry  Operator=cos
  cos : Outport  VectorParamsAs1DForOutWhenUnconnected=off
  wires:
  Trigonometric Function/1 -> cos/1
  Constant/1 -> Trigonometric Function/1

== system MPG_MG_PLL_orig/Voltage Source Inverter 4/CDSC-PLL/DSC2/DSC_Beta/Sin 2*pi//n ==
  note: 2*pi/n
  Constant : Constant  Value=2*pi/n
  Trigonometric Function : Trigonometry
  sin : Outport  VectorParamsAs1DForOutWhenUnconnected=off
  wires:
  Trigonometric Function/1 -> sin/1
  Constant/1 -> Trigonometric Function/1

== system MPG_MG_PLL_orig/Voltage Source Inverter 4/CDSC-PLL/DSC2/DSC_alpha/Cos 2*pi//n ==
  note: 2*pi*hr/n
  Constant : Constant  Value=2*pi/n
  Trigonometric Function : Trigonometry  Operator=cos
  cos : Outport  VectorParamsAs1DForOutWhenUnconnected=off
  wires:
  Trigonometric Function/1 -> cos/1
  Constant/1 -> Trigonometric Function/1

== system MPG_MG_PLL_orig/Voltage Source Inverter 4/CDSC-PLL/DSC2/DSC_alpha/Sin 2*pi//n ==
  note: 2*pi/n
  Constant : Constant  Value=2*pi/n
  Trigonometric Function : Trigonometry
  sin : Outport  VectorParamsAs1DForOutWhenUnconnected=off
  wires:
  Trigonometric Function/1 -> sin/1
  Constant/1 -> Trigonometric Function/1

== system MPG_MG_PLL_orig/Voltage Source Inverter 4/CDSC-PLL/DSC4/DSC_Beta/Cos 2*pi//n ==
  note: 2*pi*hr/n
  Constant : Constant  Value=2*pi/n
  Trigonometric Function : Trigonometry  Operator=cos
  cos : Outport  VectorParamsAs1DForOutWhenUnconnected=off
  wires:
  Trigonometric Function/1 -> cos/1
  Constant/1 -> Trigonometric Function/1

== system MPG_MG_PLL_orig/Voltage Source Inverter 4/CDSC-PLL/DSC4/DSC_Beta/Sin 2*pi//n ==
  note: 2*pi/n
  Constant : Constant  Value=2*pi/n
  Trigonometric Function : Trigonometry
  sin : Outport  VectorParamsAs1DForOutWhenUnconnected=off
  wires:
  Trigonometric Function/1 -> sin/1
  Constant/1 -> Trigonometric Function/1

== system MPG_MG_PLL_orig/Voltage Source Inverter 4/CDSC-PLL/DSC4/DSC_alpha/Cos 2*pi//n ==
  note: 2*pi*hr/n
  Constant : Constant  Value=2*pi/n
  Trigonometric Function : Trigonometry  Operator=cos
  cos : Outport  VectorParamsAs1DForOutWhenUnconnected=off
  wires:
  Trigonometric Function/1 -> cos/1
  Constant/1 -> Trigonometric Function/1

== system MPG_MG_PLL_orig/Voltage Source Inverter 4/CDSC-PLL/DSC4/DSC_alpha/Sin 2*pi//n ==
  note: 2*pi/n
  Constant : Constant  Value=2*pi/n
  Trigonometric Function : Trigonometry
  sin : Outport  VectorParamsAs1DForOutWhenUnconnected=off
  wires:
  Trigonometric Function/1 -> sin/1
  Constant/1 -> Trigonometric Function/1

== system MPG_MG_PLL_orig/Voltage Source Inverter 4/CDSC-PLL/DSC8/DSC_Beta/Cos 2*pi//n ==
  note: 2*pi*hr/n
  Constant : Constant  Value=2*pi/n
  Trigonometric Function : Trigonometry  Operator=cos
  cos : Outport  VectorParamsAs1DForOutWhenUnconnected=off
  wires:
  Trigonometric Function/1 -> cos/1
  Constant/1 -> Trigonometric Function/1

== system MPG_MG_PLL_orig/Voltage Source Inverter 4/CDSC-PLL/DSC8/DSC_Beta/Sin 2*pi//n ==
  note: 2*pi/n
  Constant : Constant  Value=2*pi/n
  Trigonometric Function : Trigonometry
  sin : Outport  VectorParamsAs1DForOutWhenUnconnected=off
  wires:
  Trigonometric Function/1 -> sin/1
  Constant/1 -> Trigonometric Function/1

== system MPG_MG_PLL_orig/Voltage Source Inverter 4/CDSC-PLL/DSC8/DSC_alpha/Cos 2*pi//n ==
  note: 2*pi*hr/n
  Constant : Constant  Value=2*pi/n
  Trigonometric Function : Trigonometry  Operator=cos
  cos : Outport  VectorParamsAs1DForOutWhenUnconnected=off
  wires:
  Trigonometric Function/1 -> cos/1
  Constant/1 -> Trigonometric Function/1

== system MPG_MG_PLL_orig/Voltage Source Inverter 4/CDSC-PLL/DSC8/DSC_alpha/Sin 2*pi//n ==
  note: 2*pi/n
  Constant : Constant  Value=2*pi/n
  Trigonometric Function : Trigonometry
  sin : Outport  VectorParamsAs1DForOutWhenUnconnected=off
  wires:
  Trigonometric Function/1 -> sin/1
  Constant/1 -> Trigonometric Function/1

== system MPG_MG_PLL_orig/Voltage Source Inverter 5/CDSC-PLL/DSC16/DSC_Beta/Cos 2*pi//n ==
  note: 2*pi*hr/n
  Constant : Constant  Value=2*pi/n
  Trigonometric Function : Trigonometry  Operator=cos
  cos : Outport  VectorParamsAs1DForOutWhenUnconnected=off
  wires:
  Trigonometric Function/1 -> cos/1
  Constant/1 -> Trigonometric Function/1

== system MPG_MG_PLL_orig/Voltage Source Inverter 5/CDSC-PLL/DSC16/DSC_Beta/Sin 2*pi//n ==
  note: 2*pi/n
  Constant : Constant  Value=2*pi/n
  Trigonometric Function : Trigonometry
  sin : Outport  VectorParamsAs1DForOutWhenUnconnected=off
  wires:
  Trigonometric Function/1 -> sin/1
  Constant/1 -> Trigonometric Function/1

== system MPG_MG_PLL_orig/Voltage Source Inverter 5/CDSC-PLL/DSC16/DSC_alpha/Cos 2*pi//n ==
  note: 2*pi*hr/n
  Constant : Constant  Value=2*pi/n
  Trigonometric Function : Trigonometry  Operator=cos
  cos : Outport  VectorParamsAs1DForOutWhenUnconnected=off
  wires:
  Trigonometric Function/1 -> cos/1
  Constant/1 -> Trigonometric Function/1

== system MPG_MG_PLL_orig/Voltage Source Inverter 5/CDSC-PLL/DSC16/DSC_alpha/Sin 2*pi//n ==
  note: 2*pi/n
  Constant : Constant  Value=2*pi/n
  Trigonometric Function : Trigonometry
  sin : Outport  VectorParamsAs1DForOutWhenUnconnected=off
  wires:
  Trigonometric Function/1 -> sin/1
  Constant/1 -> Trigonometric Function/1

== system MPG_MG_PLL_orig/Voltage Source Inverter 5/CDSC-PLL/DSC2/DSC_Beta/Cos 2*pi//n ==
  note: 2*pi*hr/n
  Constant : Constant  Value=2*pi/n
  Trigonometric Function : Trigonometry  Operator=cos
  cos : Outport  VectorParamsAs1DForOutWhenUnconnected=off
  wires:
  Trigonometric Function/1 -> cos/1
  Constant/1 -> Trigonometric Function/1

== system MPG_MG_PLL_orig/Voltage Source Inverter 5/CDSC-PLL/DSC2/DSC_Beta/Sin 2*pi//n ==
  note: 2*pi/n
  Constant : Constant  Value=2*pi/n
  Trigonometric Function : Trigonometry
  sin : Outport  VectorParamsAs1DForOutWhenUnconnected=off
  wires:
  Trigonometric Function/1 -> sin/1
  Constant/1 -> Trigonometric Function/1

== system MPG_MG_PLL_orig/Voltage Source Inverter 5/CDSC-PLL/DSC2/DSC_alpha/Cos 2*pi//n ==
  note: 2*pi*hr/n
  Constant : Constant  Value=2*pi/n
  Trigonometric Function : Trigonometry  Operator=cos
  cos : Outport  VectorParamsAs1DForOutWhenUnconnected=off
  wires:
  Trigonometric Function/1 -> cos/1
  Constant/1 -> Trigonometric Function/1

== system MPG_MG_PLL_orig/Voltage Source Inverter 5/CDSC-PLL/DSC2/DSC_alpha/Sin 2*pi//n ==
  note: 2*pi/n
  Constant : Constant  Value=2*pi/n
  Trigonometric Function : Trigonometry
  sin : Outport  VectorParamsAs1DForOutWhenUnconnected=off
  wires:
  Trigonometric Function/1 -> sin/1
  Constant/1 -> Trigonometric Function/1

== system MPG_MG_PLL_orig/Voltage Source Inverter 5/CDSC-PLL/DSC4/DSC_Beta/Cos 2*pi//n ==
  note: 2*pi*hr/n
  Constant : Constant  Value=2*pi/n
  Trigonometric Function : Trigonometry  Operator=cos
  cos : Outport  VectorParamsAs1DForOutWhenUnconnected=off
  wires:
  Trigonometric Function/1 -> cos/1
  Constant/1 -> Trigonometric Function/1

== system MPG_MG_PLL_orig/Voltage Source Inverter 5/CDSC-PLL/DSC4/DSC_Beta/Sin 2*pi//n ==
  note: 2*pi/n
  Constant : Constant  Value=2*pi/n
  Trigonometric Function : Trigonometry
  sin : Outport  VectorParamsAs1DForOutWhenUnconnected=off
  wires:
  Trigonometric Function/1 -> sin/1
  Constant/1 -> Trigonometric Function/1

== system MPG_MG_PLL_orig/Voltage Source Inverter 5/CDSC-PLL/DSC4/DSC_alpha/Cos 2*pi//n ==
  note: 2*pi*hr/n
  Constant : Constant  Value=2*pi/n
  Trigonometric Function : Trigonometry  Operator=cos
  cos : Outport  VectorParamsAs1DForOutWhenUnconnected=off
  wires:
  Trigonometric Function/1 -> cos/1
  Constant/1 -> Trigonometric Function/1

== system MPG_MG_PLL_orig/Voltage Source Inverter 5/CDSC-PLL/DSC4/DSC_alpha/Sin 2*pi//n ==
  note: 2*pi/n
  Constant : Constant  Value=2*pi/n
  Trigonometric Function : Trigonometry
  sin : Outport  VectorParamsAs1DForOutWhenUnconnected=off
  wires:
  Trigonometric Function/1 -> sin/1
  Constant/1 -> Trigonometric Function/1

== system MPG_MG_PLL_orig/Voltage Source Inverter 5/CDSC-PLL/DSC8/DSC_Beta/Cos 2*pi//n ==
  note: 2*pi*hr/n
  Constant : Constant  Value=2*pi/n
  Trigonometric Function : Trigonometry  Operator=cos
  cos : Outport  VectorParamsAs1DForOutWhenUnconnected=off
  wires:
  Trigonometric Function/1 -> cos/1
  Constant/1 -> Trigonometric Function/1

== system MPG_MG_PLL_orig/Voltage Source Inverter 5/CDSC-PLL/DSC8/DSC_Beta/Sin 2*pi//n ==
  note: 2*pi/n
  Constant : Constant  Value=2*pi/n
  Trigonometric Function : Trigonometry
  sin : Outport  VectorParamsAs1DForOutWhenUnconnected=off
  wires:
  Trigonometric Function/1 -> sin/1
  Constant/1 -> Trigonometric Function/1

== system MPG_MG_PLL_orig/Voltage Source Inverter 5/CDSC-PLL/DSC8/DSC_alpha/Cos 2*pi//n ==
  note: 2*pi*hr/n
  Constant : Constant  Value=2*pi/n
  Trigonometric Function : Trigonometry  Operator=cos
  cos : Outport  VectorParamsAs1DForOutWhenUnconnected=off
  wires:
  Trigonometric Function/1 -> cos/1
  Constant/1 -> Trigonometric Function/1

== system MPG_MG_PLL_orig/Voltage Source Inverter 5/CDSC-PLL/DSC8/DSC_alpha/Sin 2*pi//n ==
  note: 2*pi/n
  Constant : Constant  Value=2*pi/n
  Trigonometric Function : Trigonometry
  sin : Outport  VectorParamsAs1DForOutWhenUnconnected=off
  wires:
  Trigonometric Function/1 -> sin/1
  Constant/1 -> Trigonometric Function/1

== matlab function MPG_MG_PLL_orig/Voltage Source Inverter 2/Model Predictive Control  ==
  settings: updateMethod=DISCRETE  sampleTime=Ts
  data: S_opt output; Sopt output size=[1 6]; Vc input; i_filter input; vref input; Vi_opt output; Vdc parameter double size=1; modT parameter size=1; Cfilter parameter size=1; Lfilter parameter size=1
function [S_opt, Sopt, Vi_opt] = MPC(Vc, i_filter,vref,Vdc,modT,Cfilter,Lfilter)

    % In order to call "cont2dis" function
    coder.extrinsic('cont2dis');
    persistent Aq Bq Bdq Vck ifk  Vc_old if_old x_opt g f_window f_window2

    % Initialize variables and get the parameters of the Discrete model based on Ts
    if isempty(x_opt), x_opt = ones(1, 2); end
    if isempty(Vc_old), Vc_old = 0 + 1j*0; end
    if isempty(if_old), if_old = 0 + 1j*0; end
    if isempty(Vck), Vck = ones(1, 4) * (0 + 1j*0); end
    if isempty(ifk), ifk = ones(1, 4) * (0 + 1j*0); end
    if isempty(f_window), f_window = zeros(1,51); end
    if isempty(f_window2), f_window2 = zeros(1,51); end

    if isempty(Aq) && isempty(Bq) && isempty(Bdq)
        Aq = zeros(2);     Bq = zeros(2,1);     Bdq = zeros(2,1);
        % Call "cont2dis" function
        [Aq, Bq, Bdq] = cont2dis(modT,Lfilter,Cfilter); 
    end
    
    % Intialize the cost function
    g_opt = inf;
    
    % To generate the switching states matrix
    states = [1 0 0;
              0 0 0  
              1 1 0
              0 1 0
              0 1 1
              0 0 1
              1 0 1
              1 1 1];
    a = exp(1j*(2*pi/3));
    % Read current measurements at sampling instant k
    ifk(1) = i_filter;
    Vck(1) = Vc;
    % Equation of io(k-1) = if(k-1)-(c/Ts)(vc(k)-vc(k-1)).
    io = ones(1, 3) * (0 + 1j*0);
    io(1) = if_old - (Cfilter/modT)*(Vck(1) - Vc_old); 
    
    % Store the measured current for the next iteration
    if_old = i_filter;
    Vc_old = Vc;
    % FOR loop to find the best switch in the next instant and its corresponding V(i)
    k = ones(1,3);
    s = zeros(3,3);
    sw = zeros(1,3)* (0 + 1j*0);
    Vi = zeros(1,3)* (0 + 1j*0);
    for a1 = 1:8
        k(1) = a1;
        %constraint check
        if (abs(states(k(1),:)-states(x_opt(1),:)) > 1)
            continue
        end
        %state calculation
        s(1,:) = states(k(1),:);
        sw(1) = (2/3)*(s(1,1)+a*s(1,2)+a^2*s(1,3));
        Vi(1) = Vdc*sw(1);

        % Output Voltage Prediction at instant k+1
        ifk(2) = Aq(1,1)*ifk(1) + Aq(1,2)*Vck(1) + Bq(1)*Vi(1) + Bdq(1)*io(1); 
        Vck(2) = Aq(2,1)*ifk(1) + Aq(2,2)*Vck(1) + Bq(2)*Vi(1) + Bdq(2)*io(1); 
        
        for a2 = 1:8
            k(2) = a2;
            %constraint check
            if (abs(states(k(2),:)-states(k(1),:)) > 1)
                continue
            end
            io(2) = io(1) - (Cfilter/modT)*(Vck(2) - Vck(1));
            %state calculation
            s(2,:) = states(k(2),:);
            sw(2) = (2/3)*(s(2,1)+a*s(2,2)+a^2*s(2,3));
            Vi(2) = Vdc*sw(2);
    
            % Output Voltage Prediction at instant k+1
            ifk(3) = Aq(1,1)*ifk(2) + Aq(1,2)*Vck(2) + Bq(1)*Vi(2) + Bdq(1)*io(2); 
            Vck(3) = Aq(2,1)*ifk(2) + Aq(2,2)*Vck(2) + Bq(2)*Vi(2) + Bdq(2)*io(2); 

            g1 = (real(ifk(3))-real(io(3))+Cfilter*2*pi*50*imag(vref))^2 + (imag(ifk(3))-imag(io(3))+Cfilter*2*pi*50*real(vref))^2;
            g = (real(vref)-real(Vck(3)))^2+(imag(vref)-imag(Vck(3)))^2 + 0.1*g1 + 0.05*sum(states(a2)-states(a1),'all')^2;
            if (g<g_opt)
                x_opt = [k(1) k(2)];
                g_opt = g;
            end
           
        end 
    end

     
    
    % Output switching states and its voltage vector. 
    Vi_opt = x_opt(1); 
    S_opt = states(x_opt(1),:);
    d_opt = not(S_opt);
    Sopt = [S_opt,d_opt];     

end
